simulink model "mymodel"  (R2023b)
settings: Solver=VariableStepAuto  StartTime=0.0  StopTime=T  RelTol=1e-3
values from neighbouring files (symbols this model uses):
  t_gap = evalin('base', 't_gap')    [AccLogic.m]    (also in AdaptiveCruiseControlExample.m = 1.4; main.m = 1.4; matlab.mat = 1.4; test2.m)
  Ts = evalin('base', 'Ts')    [AccLogic.m]    (also in AdaptiveCruiseControlExample.m = 0.1; main.m = 0.1; matlab.mat = 0.1; test2.m)
  v0_ego = evalin('base', 'v0_ego')    [AccLogic.m]    (also in AdaptiveCruiseControlExample.m = 20; main.m = 20; matlab.mat = 20; test2.m)
  v0_lead = evalin('base', 'v0_lead')    [AccLogic.m]    (also in AdaptiveCruiseControlExample.m = 25; main.m = 25; matlab.mat = 25; test2.m = 25)
  v_set = evalin('base', 'v_set')    [AccLogic.m]    (also in AdaptiveCruiseControlExample.m = 20; main.m = 30; matlab.mat = 27.6907; test2.m)
  x0_ego = evalin('base', 'x0_ego')    [AccLogic.m]    (also in AdaptiveCruiseControlExample.m = 10; main.m = 10; matlab.mat = 10; test2.m)
  x0_lead = evalin('base', 'x0_lead')    [AccLogic.m]    (also in AdaptiveCruiseControlExample.m = 50; main.m = 50; matlab.mat = 50; test2.m)
libraries: mpcadaslib x1
settings Model: Creator=yedhukrishna  LastModifiedBy=yedhukrishna

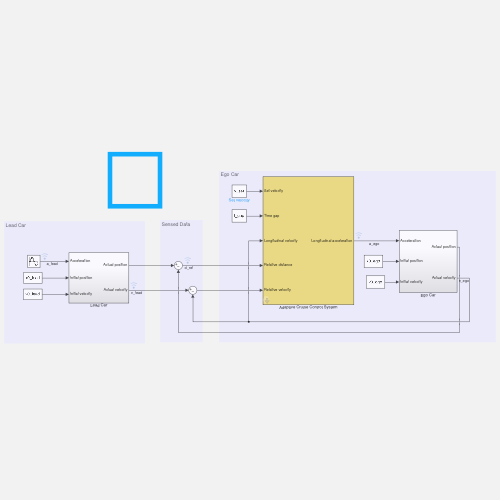
[thumbnail: Simulink's stored preview of the top-level diagram]
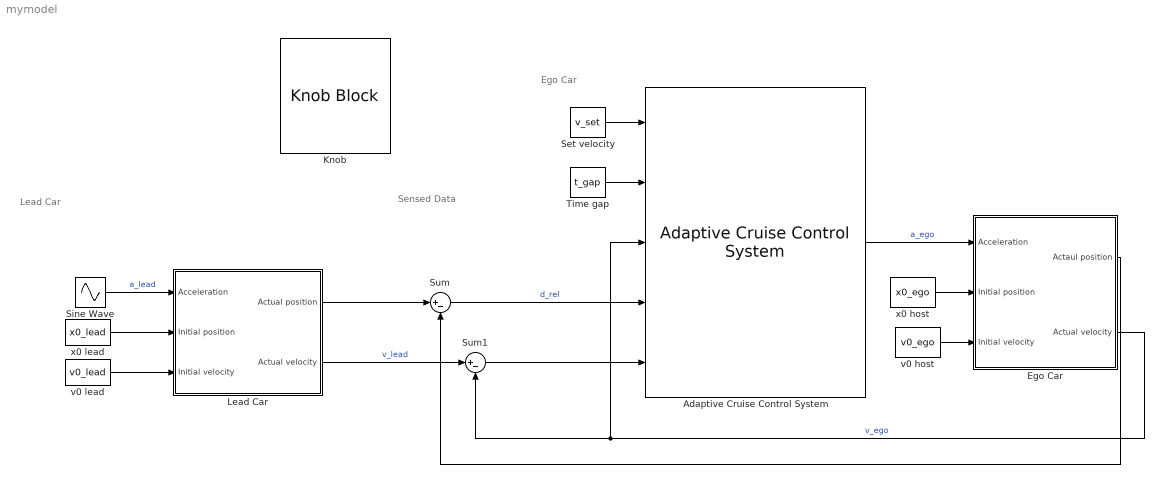
== system mymodel ==
  note: Ego Car
  note: Sensed Data
  note: Lead Car
  Adaptive Cruise Control System : mpcadaslib/Adaptive Cruise Control System  EgoModel=tf(1,[0.5,1,0])  InitialEgoVelocity=20  DefaultSpacing=10  MaxVelocity=50  MinAcceleration=-3  amin_ext=off  MaxAcceleration=2  amax_ext=off  Ts=0.1  PredictionHorizon=30  ControllerBehavior=0.5  suboptimal=off  maxiter=10  datatypeopt=double  optmode=off  trackmode=off
  Ego Car : Subsystem
  Knob : KnobBlock
  Lead Car : Subsystem
  Set velocity : Constant  Value=v_set  SampleTime=Ts
  Sine Wave : Sin  Amplitude=0.6  Frequency=0.2  SampleTime=Ts
  Sum : Sum  Inputs=|+-
  Sum1 : Sum  Inputs=|+-
  Time gap : Constant  Value=t_gap  SampleTime=Ts
  v0 host : Constant  Value=v0_ego  SampleTime=Ts
  v0 lead : Constant  Value=v0_lead  SampleTime=Ts
  x0 host : Constant  Value=x0_ego  SampleTime=Ts
  x0 lead : Constant  Value=x0_lead  SampleTime=Ts
  wires:
  x0 host/1 -> Ego Car/2(Initial position)
  v0 lead/1 -> Lead Car/3(Initial velocity)
  Ego Car/1(Actaul position) -> Sum/2
  x0 lead/1 -> Lead Car/2(Initial position)
  Sum/1 -> Adaptive Cruise Control System/4  "d_rel"
  Time gap/1 -> Adaptive Cruise Control System/2
  Lead Car/2(Actual velocity) -> Sum1/1  "v_lead"
  Ego Car/2(Actual velocity) -> Adaptive Cruise Control System/3, Sum1/2  "v_ego"
  Sine Wave/1 -> Lead Car/1(Acceleration)  "a_lead"
  Sum1/1 -> Adaptive Cruise Control System/5
  v0 host/1 -> Ego Car/3(Initial velocity)
  Set velocity/1 -> Adaptive Cruise Control System/1
  Adaptive Cruise Control System/1 -> Ego Car/1(Acceleration)  "a_ego"
  Lead Car/1(Actual position) -> Sum/1

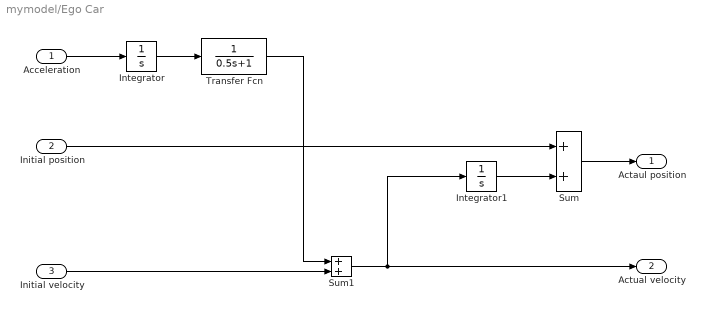
== system mymodel/Ego Car ==
  Acceleration : Inport
  Initial position : Inport  Port=2
  Initial velocity : Inport  Port=3
  Integrator : Integrator  UpperSaturationLimit=49.6351
  Integrator1 : Integrator
  Sum : Sum
  Sum1 : Sum
  Transfer Fcn : TransferFcn  Denominator=[0.5 1]
  Actaul position : Outport  VectorParamsAs1DForOutWhenUnconnected=off
  Actual velocity : Outport  Port=2  VectorParamsAs1DForOutWhenUnconnected=off
  wires:
  Integrator1/1 -> Sum/2
  Integrator/1 -> Transfer Fcn/1
  Acceleration/1 -> Integrator/1
  Sum1/1 -> Integrator1/1, Actual velocity/1
  Initial position/1 -> Sum/1
  Transfer Fcn/1 -> Sum1/1
  Sum/1 -> Actaul position/1
  Initial velocity/1 -> Sum1/2

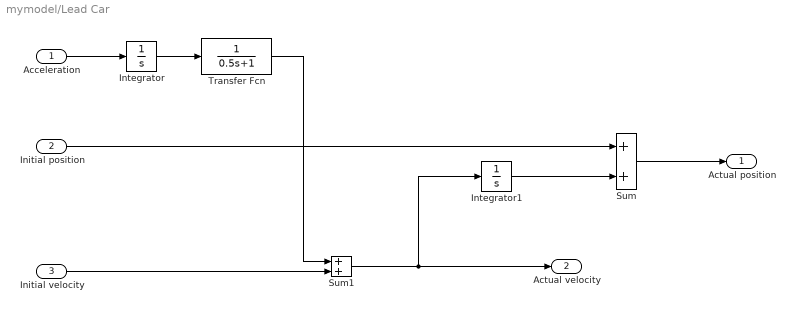
== system mymodel/Lead Car ==
  Acceleration : Inport
  Initial position : Inport  Port=2
  Initial velocity : Inport  Port=3
  Integrator : Integrator
  Integrator1 : Integrator
  Sum : Sum
  Sum1 : Sum
  Transfer Fcn : TransferFcn  Denominator=[0.5 1]
  Actual position : Outport  VectorParamsAs1DForOutWhenUnconnected=off
  Actual velocity : Outport  Port=2  VectorParamsAs1DForOutWhenUnconnected=off
  wires:
  Transfer Fcn/1 -> Sum1/1
  Initial velocity/1 -> Sum1/2
  Sum/1 -> Actual position/1
  Integrator/1 -> Transfer Fcn/1
  Sum1/1 -> Integrator1/1, Actual velocity/1
  Acceleration/1 -> Integrator/1
  Initial position/1 -> Sum/1
  Integrator1/1 -> Sum/2
